simulink model "att_controller"  (R2021b)
settings: Solver=VariableStepAuto  StartTime=0.0  StopTime=10.0  RelTol=1e-3
settings Model: Creator=aoa  LastModifiedBy=aoa

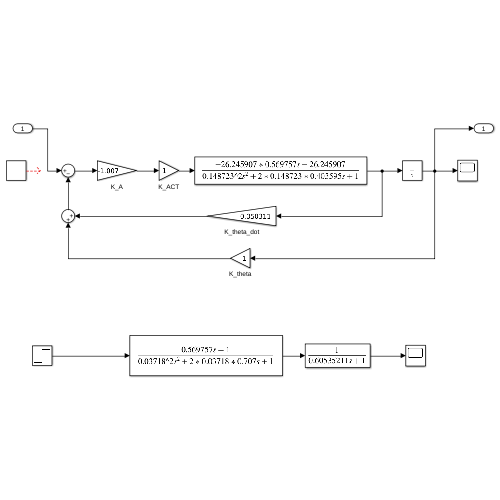
[thumbnail: Simulink's stored preview of the top-level diagram]
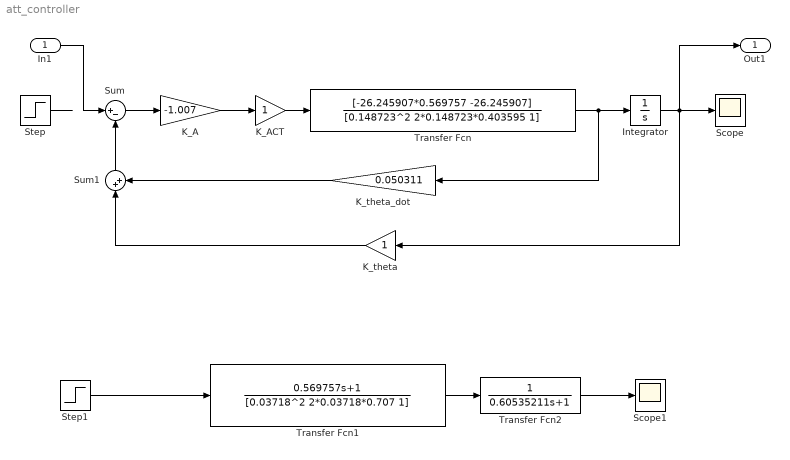
== system att_controller ==
  In1 : Inport
  Integrator : Integrator
  K_A : Gain  Gain=-1.007
  K_ACT : Gain
  K_theta : Gain
  K_theta_dot : Gain  Gain=0.050311
  Scope : Scope
  Scope1 : Scope
  Step : Step  SampleTime=0
  Step1 : Step  SampleTime=0
  Sum : Sum  Inputs=|+-
  Sum1 : Sum  Inputs=|++
  Transfer Fcn : TransferFcn  Numerator=[-26.245907*0.569757 -26.245907]  Denominator=[0.148723^2 2*0.148723*0.403595 1]
  Transfer Fcn1 : TransferFcn  Numerator=[0.569757 1]  Denominator=[0.03718^2 2*0.03718*0.707 1]
  Transfer Fcn2 : TransferFcn  Denominator=[0.60535211 1]
  Out1 : Outport
  wires:
  Step/1 -> ?
  Sum/1 -> K_A/1
  K_A/1 -> K_ACT/1
  K_ACT/1 -> Transfer Fcn/1
  Transfer Fcn/1 -> K_theta_dot/1, Integrator/1
  Integrator/1 -> Out1/1, K_theta/1, Scope/1
  K_theta_dot/1 -> Sum1/2
  K_theta/1 -> Sum1/1
  Sum1/1 -> Sum/2
  Transfer Fcn1/1 -> Transfer Fcn2/1
  Transfer Fcn2/1 -> Scope1/1
  In1/1 -> Sum/1
  Step1/1 -> Transfer Fcn1/1
